simulink model "AbstractFuelControl_M1_FP"  (R2013a)
settings: Solver=ode15s  SolverMode=SingleTasking  StartTime=0  StopTime=simTime  FixedStep=1e-04  RelTol=1e-06  AbsTol=1e-06
values from neighbouring files (symbols this model uses):
  AF_sensor_tol = 1.0    (= 1)    [AbstractFuelControl.m]    (also in AbstractFuelControl_BB.m; AbstractFuelControl_FR.m)
  fault_time = 60    [AbstractFuelControl.m]    (also in AbstractFuelControl_BB.m; AbstractFuelControl_FR.m)
  fuel_inj_tol = 1.0    (= 1)    [AbstractFuelControl.m]    (also in AbstractFuelControl_BB.m; AbstractFuelControl_FR.m)
  MAF_sensor_tol = 1.0    (= 1)    [AbstractFuelControl.m]    (also in AbstractFuelControl_BB.m; AbstractFuelControl_FR.m)
  measureTime = 1    [AbstractFuelControl.m]    (also in AbstractFuelControl_BB.m; AbstractFuelControl_FR.m)
  simTime = 50    [AbstractFuelControl.m]    (also in AbstractFuelControl_BB.m = 15; AbstractFuelControl_FR.m = 12)
  spec_num = 1    [AbstractFuelControl.m]    (also in AbstractFuelControl_BB.m; AbstractFuelControl_FR.m)
(part 1 of 2)
Description:
  | Modeling Engine Timing Using Triggered Subsystems
  | 
  | This example presents a model of a four-cylinder spark ignition engine
  | and demonstrates Simulink(R) capabilities to model an internal combustion
  | engine from the throttle to the crankshaft output. We used well-defined
  | physical principles supplemented, where appropriate, with empirical
  | relationships that describe the systems dynamic behavior without
  | introducing unnecessary complexity.
settings Model: CovMetricSettings=d  ExtModeTrigMode=oneshot  ExtModeArmWhenConnect=off  ExtModeAutoUpdateStatusClock=off  Creator=The MathWorks Inc.  LastModifiedBy=zutshi
settings SolverCC: ConsecutiveZCsStepRelTol=2.8421709430404e-13
settings DataIOCC: ExternalInput=[simTime, en_speed]  InitialState=[]  LimitDataPoints=off  LoadExternalInput=on  SignalLoggingSaveFormat=ModelDataLogs  SaveOutput=off  SignalLogging=off  SaveTime=off  StateSaveName=x  TimeSaveName=t  OutputSaveName=y  SignalLoggingName=sldemo_engine_output
settings OptimizationCC: BlockReduction=off  BooleanDataType=off  ExpressionDepthLimit=2147483647  InitFltsAndDblsToZero=on  OptimizeModelRefInitCode=on  LifeSpan=1  BufferReusableBoundary=off
settings DebuggingCC: SignalInfNanChecking=warning  SaveWithParameterizedLinksMsg=none  SignalResolutionControl=TryResolveAllWithWarning  SolverPrmCheckMsg=none  InheritedTsInSrcMsg=none  MultiTaskDSMMsg=warning  MultiTaskCondExecSysMsg=none  SigSpecEnsureSampleTimeMsg=none  IntegerOverflowMsg=none  ParameterPrecisionLossMsg=none  FcnCallInpInsideContextMsg=UseLocalSettings  UniqueDataStoreMsg=warning  StrictBusMsg=None
settings RTWCC: SystemTargetFile=ert.tlc  TemplateMakefile=ert_default_tmf  Description=Embedded Coder  GenerateReport=on  ProcessScript=ert_make_rtw_hook  IncludeHyperlinkInReport=on  IncludeERTFirstTime=on  GenerateTraceInfo=on  GenerateWebview=on
settings CodeAppCC: IgnoreCustomStorageClasses=off
settings ERTTargetCC: IncludeMdlTerminateFcn=off  MultiInstanceERTCode=on  SupportNonFinite=off  SupportComplex=off  PurelyIntegerCode=on  InlinedParameterPlacement=Hierarchical  ERTCustomFileTemplate=example_file_process.tlc  SuppressUnreachableDefaultCases=on

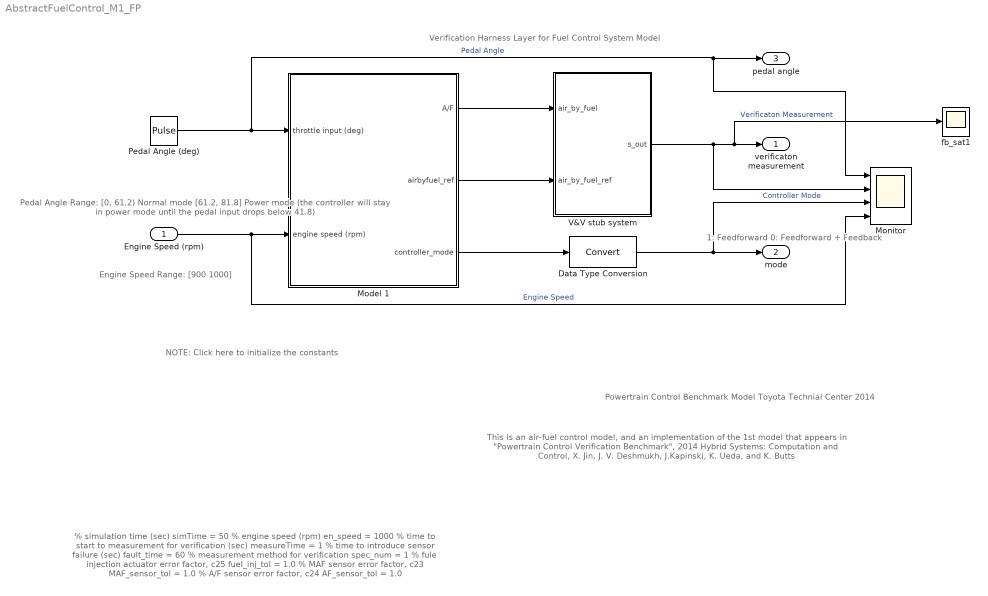
== system AbstractFuelControl_M1_FP ==
  note: 1: Feedforward
      | 0: Feedforward + Feedback
  note: NOTE: Click here to initialize the constants
  note: Pedal Angle Range:
      | [0, 61.2) Normal mode
      | [61.2, 81.8] Power mode (the controller will
      |                    stay in power mode until the pedal
      |                    input drops below 41.8)
  note: This is an air-fuel control model, and an implementation of the 1st model that appears in
      | "Powertrain Control Verification Benchmark", 2014 Hybrid Systems: Computation and Control,
      | X. Jin, J. V. Deshmukh, J.Kapinski, K. Ueda, and K. Butts
  note: % simulation time (sec)
      |     simTime = 50
      | % engine speed (rpm)
      |     en_speed = 1000
      | % time to start to measurement for verification (sec)
      |     measureTime = 1
      | % time to introduce sensor failure (sec)
      |     fault_time = 60
      | % measurement method for verification
      |     spec_num = 1
      | % fule injection actuator error factor, c25
      |     fuel_inj_tol = 1.0
      | % MAF sensor error factor, c23
      |     MAF_sensor_tol = 1.0
      | % A/F sensor error factor, c24
      |     AF_sensor_tol = 1.0
  note: Engine Speed Range:
      | [900 1000]
  note: Powertrain Control Benchmark Model
      | Toyota Technial Center
      | 2014
  note: Verification Harness Layer for Fuel Control System Model
  Engine Speed (rpm) : Inport
  Data Type Conversion : DataTypeConversion
  Model 1 : Subsystem  Priority=1  TreatAsAtomicUnit=on
  "Monitor " : Scope  NumInputPorts=4
      settings: TimeRange=30  YMin=0~-0.15~0~1000  YMax=65~0.175~1~1000
  Pedal Angle (deg) : DiscretePulseGenerator  PulseType=Time based  Amplitude=62  Period=5  PulseWidth=50
  V&V stub system : Subsystem  TreatAsAtomicUnit=on
  fb_sat1 : Scope
      settings: TimeRange=50  YMin=-0.9999  YMax=-0.999899  SaveName=ScopeData26
  verificaton measurement : Outport
  mode : Outport  Port=2
  pedal angle : Outport  Port=3
  wires:
  V&V stub system/1("s_out ") -> "Monitor "/2, fb_sat1/1, verificaton measurement/1  "Verificaton Measurement"
  Model 1/1(A/F) -> V&V stub system/1("air_by_fuel ")
  Engine Speed (rpm)/1 -> "Monitor "/4, Model 1/2(engine speed (rpm))  "Engine Speed"
  Pedal Angle (deg)/1 -> "Monitor "/1, pedal angle/1, Model 1/1(throttle input (deg))  "Pedal Angle"
  Model 1/3(controller_mode) -> Data Type Conversion/1
  Data Type Conversion/1 -> "Monitor "/3, mode/1  "Controller Mode"
  Model 1/2(airbyfuel_ref) -> V&V stub system/2(air_by_fuel_ref)

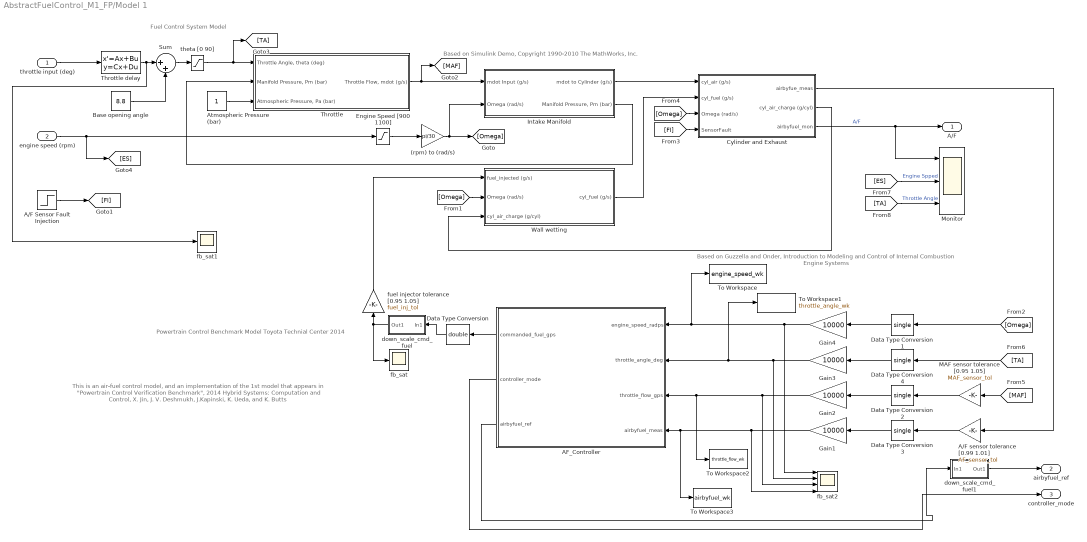
== system AbstractFuelControl_M1_FP/Model 1 ==
  note: Based on Simulink Demo, Copyright 1990-2010 The MathWorks, Inc.
  note: Based on Guzzella and Onder, Introduction to Modeling and Control of Internal Combustion Engine Systems
  note: Fuel Control System Model
  note: This is an air-fuel control model, and an implementation of the 1st model that appears in
      | "Powertrain Control Verification Benchmark", 2014 Hybrid Systems: Computation and Control,
      | X. Jin, J. V. Deshmukh, J.Kapinski, K. Ueda, and K. Butts
  note: Powertrain Control Benchmark Model
      | Toyota Technial Center
      | 2014
  throttle input (deg) : Inport  Description=[0, 81.2]
      settings: AttributesFormatString=%<Description>
  engine speed (rpm) : Inport  Description=[900,1100]  Port=2
      settings: AttributesFormatString=%<Description>
  (rpm) to (rad/s) : Gain  Gain=pi/30
  A/F Sensor Fault Injection : Step  Time=fault_time  SampleTime=0
      settings: AttributesFormatString=1: Failure\n0: Normal
  A/F sensor tolerance [0.99 1.01] : Gain  Gain=AF_sensor_tol
  AF_Controller : Subsystem  TreatAsAtomicUnit=on  SystemSampleTime=0.01
  Atmospheric Pressure (bar) : Constant
  Base opening angle : Constant  Value=8.8
  Cylinder and Exhaust : Subsystem
  Data Type Conversion : DataTypeConversion  OutDataTypeStr=double
  Data Type Conversion{1..4} (4 alike) : DataTypeConversion  OutDataTypeStr=single
  Engine Speed [900 1100] : Saturate  UpperLimit=1100  LowerLimit=900
  Gain1 : Gain  Gain=10000  ParamDataTypeStr=int32  OutDataTypeStr=Inherit: Inherit via back propagation  RndMeth=Simplest  SaturateOnIntegerOverflow=on
      settings: AttributesFormatString=up_scale
  Gain2 : Gain  Gain=10000  ParamDataTypeStr=int32  OutDataTypeStr=int32  RndMeth=Simplest  SaturateOnIntegerOverflow=on
      settings: AttributesFormatString=up_scale
  Gain3 : Gain  Gain=10000  ParamDataTypeStr=int32  OutDataTypeStr=int32  RndMeth=Simplest  SaturateOnIntegerOverflow=on
      settings: AttributesFormatString=up_scale
  Gain4 : Gain  Gain=10000  ParamDataTypeStr=int32  OutDataTypeStr=int32  RndMeth=Simplest  SaturateOnIntegerOverflow=on
      settings: AttributesFormatString=up_scale
  Intake Manifold : Subsystem
  MAF sensor tolerance [0.95 1.05] : Gain  Gain=MAF_sensor_tol
  Monitor : Scope  NumInputPorts=3
      settings: TimeRange=85  YMin=11.75~49.7419~5  YMax=14.75~54.9779~60
  Sum : Sum  Inputs=|++
  Throttle : Subsystem
  Throttle delay : StateSpace  A=-10  C=10  D=0
  To Workspace : ToWorkspace  VariableName=engine_speed_wk  SampleTime=0.01  SaveFormat=Timeseries
  To Workspace1 : ToWorkspace  VariableName=throttle_angle_wk  SampleTime=0.01  SaveFormat=Timeseries
  To Workspace2 : ToWorkspace  VariableName=throttle_flow_wk  SampleTime=0.01  SaveFormat=Timeseries
  To Workspace3 : ToWorkspace  VariableName=airbyfuel_wk  SampleTime=0.01  SaveFormat=Timeseries
  Wall wetting : Subsystem
  down_scale_cmd_fuel : Subsystem
      settings: AttributesFormatString=%<MemberBlocks>
  down_scale_cmd_fuel1 : Subsystem
      settings: AttributesFormatString=%<MemberBlocks>
  fb_sat : Scope
      settings: TimeRange=50  YMin=0.3725  YMax=0.43  SaveName=ScopeData12
  fb_sat1 : Scope
      settings: TimeRange=50  YMin=0.3725  YMax=0.43  SaveName=ScopeData22
  fb_sat2 : Scope  NumInputPorts=4
      settings: TimeRange=0.01302246191310628  YMin=1047196~0~49866.13136574067~0  YMax=1047198~200000~63254.64409722215~200000  SaveName=ScopeData25
  fuel injector tolerance [0.95 1.05] : Gain  Gain=fuel_inj_tol
  theta [0 90] : Saturate  UpperLimit=90  LowerLimit=0
  A/F : Outport
  airbyfuel_ref : Outport  Port=2
  controller_mode : Outport  Port=3
  wires:
  (rpm) to (rad/s)/1 -> [Omega], Intake Manifold/2(Omega (rad/s))
  Data Type Conversion/1 -> down_scale_cmd_fuel/1(In1)
  theta [0 90]/1 -> Throttle/1("Throttle Angle, theta (deg)"), [TA]
  Engine Speed [900 1100]/1 -> (rpm) to (rad/s)/1
  Cylinder and Exhaust/3("airbyfuel_mon ") -> A/F/1, Monitor/1  "A/F"
  Data Type Conversion2/1 -> Gain2/1
  Data Type Conversion3/1 -> Gain1/1
  A/F sensor tolerance [0.99 1.01]/1 -> Data Type Conversion3/1
  [MAF] -> MAF sensor tolerance [0.95 1.05]/1
  Cylinder and Exhaust/1(airbyfue_meas) -> A/F sensor tolerance [0.99 1.01]/1
  Throttle/1("Throttle Flow, mdot (g/s)") -> [MAF], Intake Manifold/1(mdot Input (g/s))
  Intake Manifold/2("Manifold Pressure, Pm (bar)") -> Throttle/2("Manifold Pressure, Pm (bar)")
  Atmospheric Pressure (bar)/1 -> Throttle/3("Atmospheric Pressure, Pa (bar) ")
  Wall wetting/1(cyl_fuel (g/s)) -> Cylinder and Exhaust/2(cyl_fuel (g/s))
  Intake Manifold/1(mdot to Cylinder (g/s)) -> Cylinder and Exhaust/1(cyl_air (g/s))
  [Omega] -> Cylinder and Exhaust/3(Omega (rad/s))
  [Omega] -> Wall wetting/2(Omega (rad/s))
  Cylinder and Exhaust/2(cyl_air_charge (g/cyl)) -> Wall wetting/3(cyl_air_charge (g/cyl))
  [Omega] -> Data Type Conversion1/1
  fuel injector tolerance [0.95 1.05]/1 -> Wall wetting/1(fuel_injected (g/s))
  MAF sensor tolerance [0.95 1.05]/1 -> Data Type Conversion2/1
  Data Type Conversion1/1 -> Gain4/1
  A/F Sensor Fault Injection/1 -> [FI]
  [FI] -> Cylinder and Exhaust/4(SensorFault)
  [TA] -> Data Type Conversion4/1
  Data Type Conversion4/1 -> Gain3/1
  engine speed (rpm)/1 -> [ES], Engine Speed [900 1100]/1
  [TA] -> Monitor/3  "Throttle Angle"
  Base opening angle/1 -> Sum/2
  Sum/1 -> theta [0 90]/1
  AF_Controller/2(controller_mode) -> controller_mode/1
  AF_Controller/3(airbyfuel_ref) -> down_scale_cmd_fuel1/1(In1)
  [ES] -> Monitor/2  "Engine Spped"
  throttle input (deg)/1 -> Throttle delay/1
  Throttle delay/1 -> fb_sat1/1, Sum/1
  AF_Controller/1(commanded_fuel_gps) -> Data Type Conversion/1
  down_scale_cmd_fuel/1(Out1) -> fb_sat/1, fuel injector tolerance [0.95 1.05]/1
  Gain1/1 -> fb_sat2/4, To Workspace3/1, AF_Controller/4(airbyfuel_meas)
  Gain2/1 -> fb_sat2/3, AF_Controller/3(throttle_flow_gps), To Workspace2/1
  Gain3/1 -> fb_sat2/2, To Workspace1/1, AF_Controller/2(throttle_angle_deg)
  Gain4/1 -> To Workspace/1, AF_Controller/1(engine_speed_radps), fb_sat2/1
  down_scale_cmd_fuel1/1(Out1) -> airbyfuel_ref/1

== system AbstractFuelControl_M1_FP/V&V stub system ==
  "air_by_fuel " : Inport  OutDataTypeStr=double
  air_by_fuel_ref : Inport  Port=2
  Calcuate Error : Subsystem  Priority=20  TreatAsAtomicUnit=on
  Constant : Constant  Value=0.5
  Data Type Conversion : DataTypeConversion  OutDataTypeStr=double
  MeasureOn : Step  Time=measureTime  SampleTime=0
  Relational Operator : RelationalOperator  Operator=>  OutDataTypeStr=boolean
  spec_num : Constant  Value=spec_num  OutDataTypeStr=uint8
  "s_out " : Outport
  wires:
  Calcuate Error/1("s_out ") -> "s_out "/1
  MeasureOn/1 -> Relational Operator/1
  Constant/1 -> Relational Operator/2
  Relational Operator/1 -> Calcuate Error/Enable
  spec_num/1 -> Calcuate Error/2(spec_num)
  "air_by_fuel "/1 -> Calcuate Error/1("air_by_fuel ")
  air_by_fuel_ref/1 -> Data Type Conversion/1
  Data Type Conversion/1 -> Calcuate Error/3(air_by_fuel_ref)

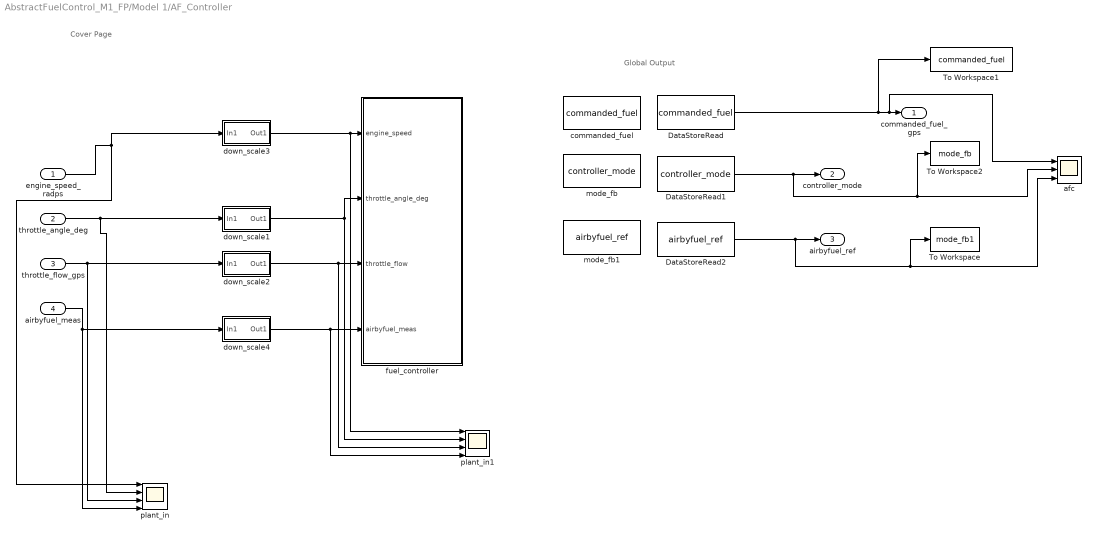
== system AbstractFuelControl_M1_FP/Model 1/AF_Controller ==
  note: Global Output
  note: Cover Page
  engine_speed_radps : Inport
  throttle_angle_deg : Inport  Port=2
  throttle_flow_gps : Inport  Port=3
  airbyfuel_meas : Inport  Port=4
  DataStoreRead : DataStoreRead  Priority=2  DataStoreName=commanded_fuel
  DataStoreRead1 : DataStoreRead  Priority=2  DataStoreName=controller_mode
  DataStoreRead2 : DataStoreRead  Priority=2  DataStoreName=airbyfuel_ref
  To Workspace : ToWorkspace  VariableName=mode_fb1  SampleTime=-1  SaveFormat=Timeseries
  To Workspace1 : ToWorkspace  VariableName=commanded_fuel  SampleTime=-1  SaveFormat=Timeseries
  To Workspace2 : ToWorkspace  VariableName=mode_fb  SampleTime=-1  SaveFormat=Timeseries
  afc : Scope  NumInputPorts=3
      settings: TimeRange=30.1  YMin=16600~-1~147  YMax=16600~1~147  SaveName=ScopeData3
  commanded_fuel : DataStoreMemory  DataStoreName=commanded_fuel  InitialValue=1726
      settings: AttributesFormatString=commanded_fuel
  down_scale1 : Subsystem
      settings: AttributesFormatString=%<MemberBlocks>
  down_scale2 : Subsystem
      settings: AttributesFormatString=%<MemberBlocks>
  down_scale3 : Subsystem
      settings: AttributesFormatString=%<MemberBlocks>
  down_scale4 : Subsystem
      settings: AttributesFormatString=%<MemberBlocks>
  fuel_controller : Subsystem  Priority=1  TreatAsAtomicUnit=on
      settings: AttributesFormatString=Priority = %<Priority>
  mode_fb : DataStoreMemory  DataStoreName=controller_mode  InitialValue=1  OutDataTypeStr=boolean
      settings: AttributesFormatString=controller_mode
  mode_fb1 : DataStoreMemory  DataStoreName=airbyfuel_ref  InitialValue=147  OutDataTypeStr=single
  plant_in : Scope  NumInputPorts=4
      settings: TimeRange=30.1  YMin=99.484~8~5~-5  YMax=109.956~19~8.25~5  SaveName=ScopeData10
  plant_in1 : Scope  NumInputPorts=4
      settings: TimeRange=30.1  YMin=98.8~8~4.75~-5  YMax=109.2~18~5.25~5  SaveName=ScopeData11
  commanded_fuel_gps : Outport
  controller_mode : Outport  Port=2
  airbyfuel_ref : Outport  Port=3
  wires:
  DataStoreRead2/1 -> To Workspace/1, afc/3, airbyfuel_ref/1
  DataStoreRead1/1 -> To Workspace2/1, afc/2, controller_mode/1
  airbyfuel_meas/1 -> down_scale4/1(In1), plant_in/4
  throttle_flow_gps/1 -> down_scale2/1(In1), plant_in/3
  throttle_angle_deg/1 -> down_scale1/1(In1), plant_in/2
  engine_speed_radps/1 -> down_scale3/1(In1), plant_in/1
  DataStoreRead/1 -> To Workspace1/1, afc/1, commanded_fuel_gps/1
  down_scale2/1(Out1) -> plant_in1/3, fuel_controller/3(throttle_flow)
  down_scale1/1(Out1) -> fuel_controller/2(throttle_angle_deg), plant_in1/2
  down_scale3/1(Out1) -> plant_in1/1, fuel_controller/1(engine_speed)
  down_scale4/1(Out1) -> plant_in1/4, fuel_controller/4(airbyfuel_meas)

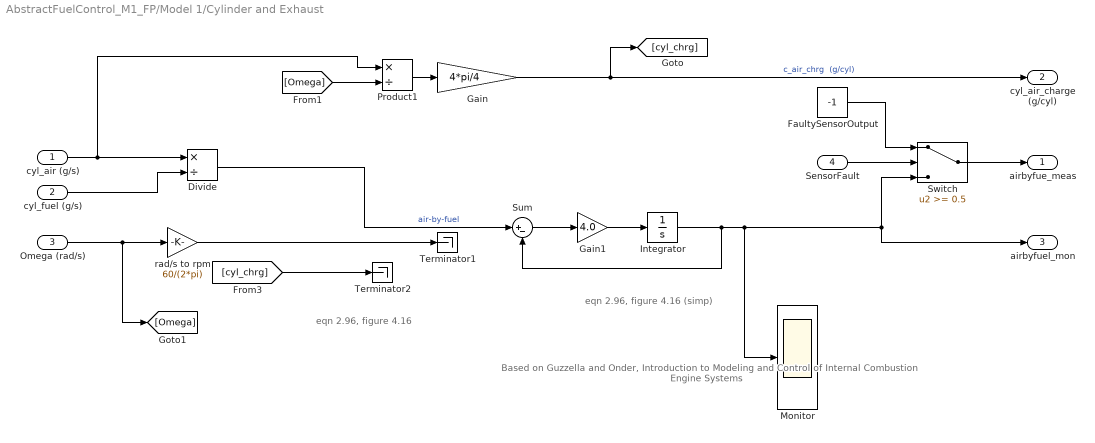
== system AbstractFuelControl_M1_FP/Model 1/Cylinder and Exhaust ==
  note: Based on Guzzella and Onder, Introduction to Modeling and Control of Internal Combustion Engine Systems
  note: eqn 2.96, figure 4.16
  note: eqn 2.96, figure 4.16 (simp)
  cyl_air (g/s) : Inport
  cyl_fuel (g/s) : Inport  Port=2
  Omega (rad/s) : Inport  Port=3
  SensorFault : Inport  Port=4
  Divide : Product  Inputs=*/
  FaultySensorOutput : Constant  Value=-1
  Gain : Gain  Gain=4*pi/4
  Gain1 : Gain  Gain=4.0
  Integrator : Integrator  ContinuousStateAttributes='cyl_ex'
  Monitor : Scope
      settings: TimeRange=85  YMin=11.75  YMax=14.75  SaveName=ScopeData21
  Product1 : Product  Inputs=*/  RndMeth=Zero
  Sum : Sum  Inputs=|+-
  Switch : Switch  Threshold=0.5
  Terminator1 : Terminator
  Terminator2 : Terminator
  rad/s to rpm : Gain  Gain=60/(2*pi)
  airbyfue_meas : Outport
  cyl_air_charge (g/cyl) : Outport  Port=2
  "airbyfuel_mon " : Outport  Port=3
  wires:
  cyl_air (g/s)/1 -> Divide/1, Product1/1
  [Omega] -> Product1/2
  Product1/1 -> Gain/1
  Gain/1 -> [cyl_chrg], cyl_air_charge (g/cyl)/1  "c_air_chrg  (g/cyl)"
  cyl_fuel (g/s)/1 -> Divide/2
  Omega (rad/s)/1 -> [Omega], rad/s to rpm/1
  Switch/1 -> airbyfue_meas/1
  FaultySensorOutput/1 -> Switch/1
  SensorFault/1 -> Switch/2
  Integrator/1 -> Monitor/1, "airbyfuel_mon "/1, Switch/3, Sum/2
  Divide/1 -> Sum/1  "air-by-fuel"
  rad/s to rpm/1 -> Terminator1/1
  [cyl_chrg] -> Terminator2/1
  Gain1/1 -> Integrator/1
  Sum/1 -> Gain1/1

== system AbstractFuelControl_M1_FP/Model 1/Intake Manifold ==
  note: Intake Manifold Vacuum
  note: Based on Simulink Demo, Copyright 1990-2010 The MathWorks, Inc.
  mdot Input (g/s) : Inport
  Omega (rad/s) : Inport  Port=2
  Gain2 : Gain  Gain=0.9  ParamDataTypeStr=single  OutDataTypeStr=Inherit: Inherit via back propagation  RndMeth=Simplest  SaturateOnIntegerOverflow=on
      settings: AttributesFormatString=pumping tolerance [0.9 1.1]
  Mux : Mux  Inputs=2
  Pumping : Fcn  Expr=-0.366 + 0.08979*u[1]*u[2] - 0.0337*u[2]*u[1]*u[1] + 0.0001*u[1]*u[2]*u[2]
  RT/Vm : Gain  Gain=0.41328  SaturateOnIntegerOverflow=on  OutDataTypeStr=Inherit: Same as input  ParamDataTypeStr=Inherit: Same as input
  Sum : Sum  Inputs=|+-  SaturateOnIntegerOverflow=on  InputSameDT=on  OutDataTypeStr=Inherit: Same as first input
  fb_sat1 : Scope
      settings: TimeRange=50  YMin=0.3725  YMax=0.43  SaveName=ScopeData23
  p0 = 0.543 (bar) : Integrator  InitialCondition=0.982  ContinuousStateAttributes='intake_manifold'
  mdot to Cylinder (g/s) : Outport  InitialOutput=0
  "Manifold Pressure, Pm (bar)" : Outport  Port=2  InitialOutput=0
  wires:
  mdot Input (g/s)/1 -> Sum/1
  RT/Vm/1 -> p0 = 0.543 (bar)/1
  Omega (rad/s)/1 -> Mux/2
  Mux/1 -> Pumping/1
  p0 = 0.543 (bar)/1 -> fb_sat1/1, Mux/1, "Manifold Pressure, Pm (bar)"/1
  Sum/1 -> RT/Vm/1
  Pumping/1 -> Gain2/1
  Gain2/1 -> Sum/2, mdot to Cylinder (g/s)/1

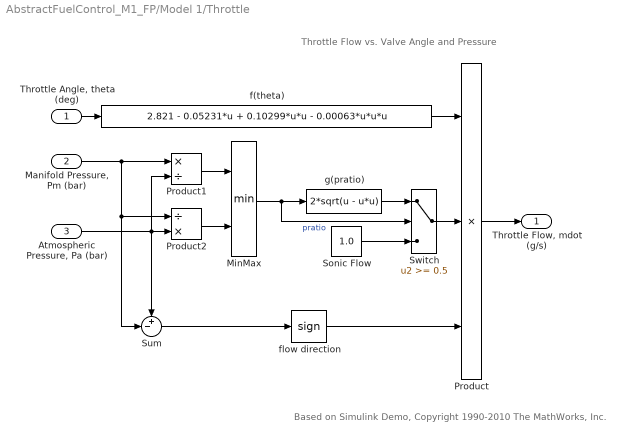
== system AbstractFuelControl_M1_FP/Model 1/Throttle ==
  note: Throttle Flow vs. Valve Angle and Pressure
  note: Based on Simulink Demo, Copyright 1990-2010 The MathWorks, Inc.
  "Throttle Angle, theta (deg)" : Inport
  "Manifold Pressure, Pm (bar)" : Inport  Port=2
  "Atmospheric Pressure, Pa (bar) " : Inport  Port=3
  MinMax : MinMax  Inputs=2  SaturateOnIntegerOverflow=on  InputSameDT=on
  Product : Product  Inputs=3  SaturateOnIntegerOverflow=on  RndMeth=Zero  InputSameDT=on  OutDataTypeStr=Inherit: Same as first input
  Product1 : Product  Inputs=*/  SaturateOnIntegerOverflow=on  RndMeth=Zero  InputSameDT=on  OutDataTypeStr=Inherit: Same as first input
  Product2 : Product  Inputs=/*  SaturateOnIntegerOverflow=on  RndMeth=Zero  InputSameDT=on  OutDataTypeStr=Inherit: Same as first input
  "Sonic Flow " : Constant  Value=1.0
  Sum : Sum  Inputs=+-|  SaturateOnIntegerOverflow=on  InputSameDT=on  OutDataTypeStr=Inherit: Same as first input
  Switch : Switch  Threshold=0.5  SaturateOnIntegerOverflow=on  InputSameDT=on
  f(theta) : Fcn  Expr=2.821 - 0.05231*u + 0.10299*u*u - 0.00063*u*u*u
  flow direction : Signum
  g(pratio) : Fcn  Expr=2*sqrt(u - u*u)
  "Throttle Flow, mdot (g/s)" : Outport  InitialOutput=0
  wires:
  "Manifold Pressure, Pm (bar)"/1 -> Sum/2, Product2/1, Product1/1
  Product2/1 -> MinMax/2
  Product1/1 -> MinMax/1
  "Atmospheric Pressure, Pa (bar) "/1 -> Sum/1, Product2/2, Product1/2
  g(pratio)/1 -> Switch/1
  "Sonic Flow "/1 -> Switch/3
  Switch/1 -> Product/2
  flow direction/1 -> Product/3
  Sum/1 -> flow direction/1
  MinMax/1 -> g(pratio)/1, Switch/2  "pratio"
  "Throttle Angle, theta (deg)"/1 -> f(theta)/1
  Product/1 -> "Throttle Flow, mdot (g/s)"/1
  f(theta)/1 -> Product/1

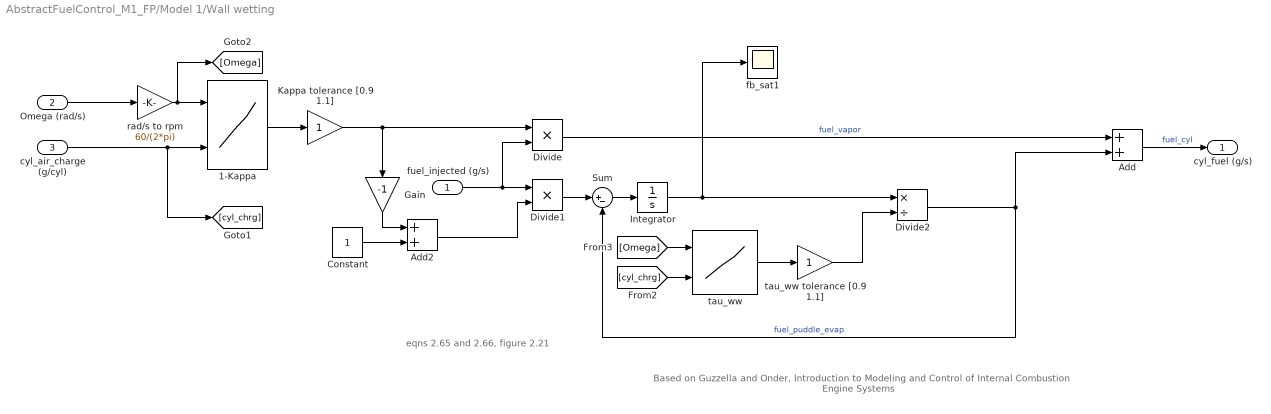
== system AbstractFuelControl_M1_FP/Model 1/Wall wetting ==
  note: Based on Guzzella and Onder, Introduction to Modeling and Control of Internal Combustion Engine Systems
  note: eqns 2.65 and 2.66, figure 2.21
  fuel_injected (g/s) : Inport
  Omega (rad/s) : Inport  Port=2
  cyl_air_charge (g/cyl) : Inport  Port=3
  1-Kappa : Lookup_n-D  BreakpointsForDimension1=[1000,1500,2000,2500,3000]  BreakpointsForDimension2=[.1,.2,.3,.4]  Table=reshape([0.8,.7,.7,.8,.9,.7,.66,.65,.73,.85,.66,.66,.63,.66,.8,.6,.6,.6,.6,.7],5,4)  UseLastTableValue=on  RndMeth=Simplest  InputSameDT=on
  Add : Sum
  Add2 : Sum
  Constant : Constant
  Divide : Product  Inputs=**
  Divide1 : Product  Inputs=**
  Divide2 : Product  Inputs=*/
  Gain : Gain  Gain=-1
  Integrator : Integrator  InitialCondition=0.0112  ContinuousStateAttributes='wall_wetting'
  Kappa tolerance [0.9 1.1] : Gain
  Sum : Sum  Inputs=|+-
  fb_sat1 : Scope
      settings: TimeRange=50  YMin=0.3725  YMax=0.43  SaveName=ScopeData24
  rad/s to rpm : Gain  Gain=60/(2*pi)
  tau_ww : Lookup_n-D  BreakpointsForDimension1=[1000,1500,2000,2500,3000]  BreakpointsForDimension2=[0.1,0.2,0.3,0.4]  Table=reshape([.4,.3,.35,.3,.2,.22,.22,.4,.35,.5,.20,.22,.5,.4,.35,.35,.3,.45,.5,.4],5,4)  UseLastTableValue=on  RndMeth=Simplest  InputSameDT=on
  tau_ww tolerance [0.9 1.1] : Gain
  cyl_fuel (g/s) : Outport
  wires:
  1-Kappa/1 -> Kappa tolerance [0.9 1.1]/1
  fuel_injected (g/s)/1 -> Divide/2, Divide1/1
  Divide/1 -> Add/1  "fuel_vapor"
  Add/1 -> cyl_fuel (g/s)/1  "fuel_cyl"
  Integrator/1 -> fb_sat1/1, Divide2/1
  Divide1/1 -> Sum/1
  Sum/1 -> Integrator/1
  Divide2/1 -> Add/2, Sum/2  "fuel_puddle_evap"
  Add2/1 -> Divide1/2
  cyl_air_charge (g/cyl)/1 -> 1-Kappa/2, [cyl_chrg]
  [cyl_chrg] -> tau_ww/2
  tau_ww/1 -> tau_ww tolerance [0.9 1.1]/1
  Gain/1 -> Add2/1
  Constant/1 -> Add2/2
  rad/s to rpm/1 -> [Omega], 1-Kappa/1
  Omega (rad/s)/1 -> rad/s to rpm/1
  Kappa tolerance [0.9 1.1]/1 -> Divide/1, Gain/1
  tau_ww tolerance [0.9 1.1]/1 -> Divide2/2
  [Omega] -> tau_ww/1

== system AbstractFuelControl_M1_FP/Model 1/down_scale_cmd_fuel ==
  In1 : Inport
  Constant8 : Constant  Value=10000  OutDataTypeStr=single  SampleTime=-1
      settings: AttributesFormatString=Value = %<Value>
  Divide2 : Product  Inputs=*/  OutDataTypeStr=Inherit: Inherit via back propagation
  Out1 : Outport
  wires:
  Constant8/1 -> Divide2/2
  Divide2/1 -> Out1/1
  In1/1 -> Divide2/1

== system AbstractFuelControl_M1_FP/Model 1/down_scale_cmd_fuel1 ==
  In1 : Inport
  Constant8 : Constant  Value=10  OutDataTypeStr=single  SampleTime=-1
      settings: AttributesFormatString=Value = %<Value>
  Divide2 : Product  Inputs=*/  OutDataTypeStr=Inherit: Inherit via back propagation
  Out1 : Outport
  wires:
  Constant8/1 -> Divide2/2
  Divide2/1 -> Out1/1
  In1/1 -> Divide2/1

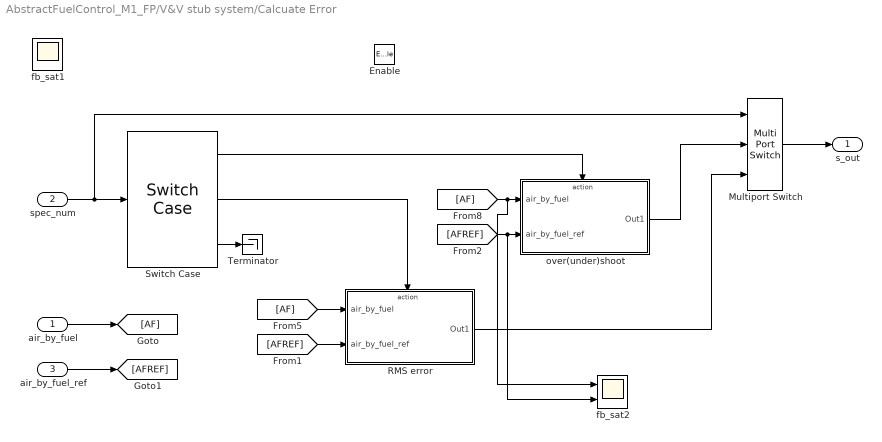
== system AbstractFuelControl_M1_FP/V&V stub system/Calcuate Error ==
  "air_by_fuel " : Inport
  spec_num : Inport  Port=2  OutDataTypeStr=uint8
  air_by_fuel_ref : Inport  Port=3
  Enable : EnablePort
  Multiport Switch : MultiPortSwitch  Inputs=2
  RMS error : Subsystem  TreatAsAtomicUnit=on
  Switch Case : SwitchCase  CaseConditions={1,2}
  Terminator : Terminator
  fb_sat1 : Scope
      settings: TimeRange=50  YMin=-0.9999  YMax=-0.999899  SaveName=ScopeData27
  fb_sat2 : Scope  NumInputPorts=2
      settings: TimeRange=50  YMin=14.425~147000  YMax=14.925~147000  SaveName=ScopeData28
  over(under)shoot : Subsystem  TreatAsAtomicUnit=on
  "s_out " : Outport
  wires:
  "air_by_fuel "/1 -> [AF]
  spec_num/1 -> Multiport Switch/1, Switch Case/1
  Switch Case/1 -> over(under)shoot/Action
  [AF] -> fb_sat2/1, over(under)shoot/1("air_by_fuel ")
  Switch Case/2 -> RMS error/Action
  [AF] -> RMS error/1("air_by_fuel ")
  Multiport Switch/1 -> "s_out "/1
  over(under)shoot/1(Out1) -> Multiport Switch/2
  RMS error/1(Out1) -> Multiport Switch/3
  Switch Case/3 -> Terminator/1
  air_by_fuel_ref/1 -> [AFREF]
  [AFREF] -> RMS error/2(air_by_fuel_ref)
  [AFREF] -> fb_sat2/2, over(under)shoot/2(air_by_fuel_ref)

== system AbstractFuelControl_M1_FP/Model 1/AF_Controller/down_scale1 ==
  In1 : Inport
  Constant8 : Constant  Value=1000  OutDataTypeStr=single  SampleTime=-1
      settings: AttributesFormatString=Value = %<Value>
  Divide2 : Product  Inputs=*/  OutDataTypeStr=Inherit: Inherit via back propagation
  Out1 : Outport
  wires:
  Constant8/1 -> Divide2/2
  Divide2/1 -> Out1/1
  In1/1 -> Divide2/1

== system AbstractFuelControl_M1_FP/Model 1/AF_Controller/down_scale2 ==
  In1 : Inport
  Constant8 : Constant  Value=1000  OutDataTypeStr=single  SampleTime=-1
      settings: AttributesFormatString=Value = %<Value>
  Divide2 : Product  Inputs=*/  OutDataTypeStr=Inherit: Inherit via back propagation
  Out1 : Outport
  wires:
  Constant8/1 -> Divide2/2
  Divide2/1 -> Out1/1
  In1/1 -> Divide2/1

== system AbstractFuelControl_M1_FP/Model 1/AF_Controller/down_scale3 ==
  In1 : Inport
  Constant8 : Constant  Value=1000  OutDataTypeStr=single  SampleTime=-1
      settings: AttributesFormatString=Value = %<Value>
  Divide2 : Product  Inputs=*/  OutDataTypeStr=Inherit: Inherit via back propagation
  Out1 : Outport
  wires:
  Constant8/1 -> Divide2/2
  Divide2/1 -> Out1/1
  In1/1 -> Divide2/1

== system AbstractFuelControl_M1_FP/Model 1/AF_Controller/down_scale4 ==
  In1 : Inport
  Constant8 : Constant  Value=1000  OutDataTypeStr=single  SampleTime=-1
      settings: AttributesFormatString=Value = %<Value>
  Divide2 : Product  Inputs=*/  OutDataTypeStr=Inherit: Inherit via back propagation
  Out1 : Outport
  wires:
  Constant8/1 -> Divide2/2
  Divide2/1 -> Out1/1
  In1/1 -> Divide2/1

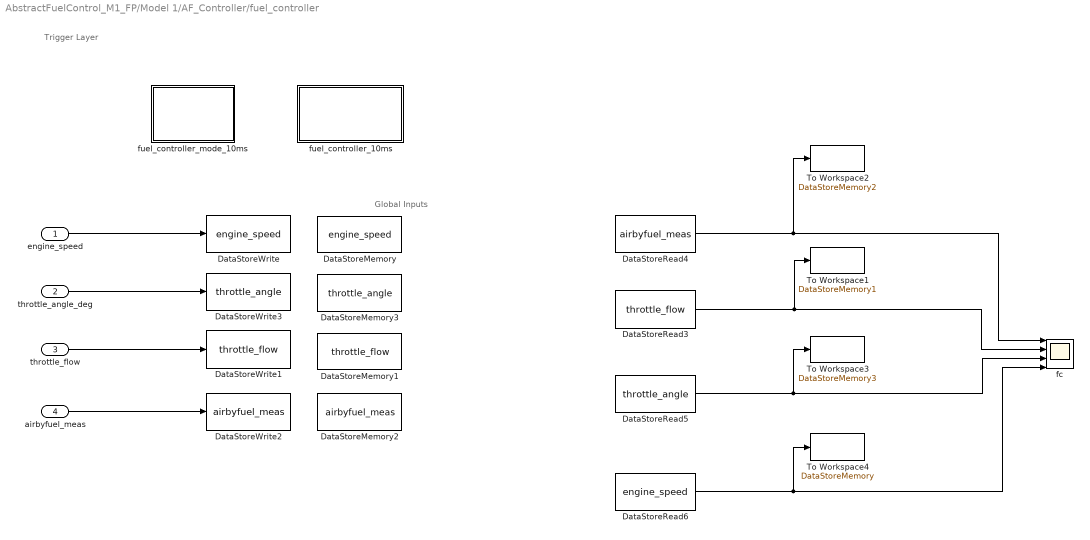
== system AbstractFuelControl_M1_FP/Model 1/AF_Controller/fuel_controller ==
  note: Global Inputs
  note: Trigger Layer
  engine_speed : Inport
  throttle_angle_deg : Inport  Port=2
  throttle_flow : Inport  Port=3
  airbyfuel_meas : Inport  Port=4
  DataStoreMemory : DataStoreMemory  DataStoreName=engine_speed  OutDataTypeStr=single
      settings: AttributesFormatString=engine speed
  DataStoreMemory1 : DataStoreMemory  DataStoreName=throttle_flow  OutDataTypeStr=single
      settings: AttributesFormatString=throttle flow
  DataStoreMemory2 : DataStoreMemory  DataStoreName=airbyfuel_meas  OutDataTypeStr=single
      settings: AttributesFormatString=lambda_meas
  DataStoreMemory3 : DataStoreMemory  DataStoreName=throttle_angle  OutDataTypeStr=single
      settings: AttributesFormatString=throttle flow
  DataStoreRead3 : DataStoreRead  DataStoreName=throttle_flow
  DataStoreRead4 : DataStoreRead  DataStoreName=airbyfuel_meas
  DataStoreRead5 : DataStoreRead  DataStoreName=throttle_angle
  DataStoreRead6 : DataStoreRead  DataStoreName=engine_speed
  DataStoreWrite : DataStoreWrite  Priority=1  DataStoreName=engine_speed
  DataStoreWrite1 : DataStoreWrite  Priority=1  DataStoreName=throttle_flow
  DataStoreWrite2 : DataStoreWrite  Priority=1  DataStoreName=airbyfuel_meas
  DataStoreWrite3 : DataStoreWrite  Priority=1  DataStoreName=throttle_angle
  To Workspace1 : ToWorkspace  VariableName=DataStoreMemory1  SampleTime=-1  SaveFormat=Timeseries
      settings: MaxDataPoints=1
  To Workspace2 : ToWorkspace  VariableName=DataStoreMemory2  SampleTime=-1  SaveFormat=Timeseries
      settings: MaxDataPoints=1
  To Workspace3 : ToWorkspace  VariableName=DataStoreMemory3  SampleTime=-1  SaveFormat=Timeseries
      settings: MaxDataPoints=1
  To Workspace4 : ToWorkspace  VariableName=DataStoreMemory  SampleTime=-1  SaveFormat=Timeseries
      settings: MaxDataPoints=1
  fc : Scope  NumInputPorts=4
      settings: TimeRange=30.1  YMin=14.5~5.5~8~99.484  YMax=15.1~8.5~19~109.956
  fuel_controller_10ms : Subsystem  Priority=30  TreatAsAtomicUnit=on
      settings: AttributesFormatString=Priority = %<Priority>
  fuel_controller_mode_10ms : Subsystem  Priority=20  TreatAsAtomicUnit=on
      settings: AttributesFormatString=Priority = %<Priority>
  wires:
  DataStoreRead4/1 -> To Workspace2/1, fc/1
  DataStoreRead3/1 -> To Workspace1/1, fc/2
  DataStoreRead5/1 -> To Workspace3/1, fc/3
  DataStoreRead6/1 -> To Workspace4/1, fc/4
  engine_speed/1 -> DataStoreWrite/1
  throttle_angle_deg/1 -> DataStoreWrite3/1
  throttle_flow/1 -> DataStoreWrite1/1
  airbyfuel_meas/1 -> DataStoreWrite2/1

== system AbstractFuelControl_M1_FP/V&V stub system/Calcuate Error/RMS error ==
  "air_by_fuel " : Inport
  air_by_fuel_ref : Inport  Port=2
  Action Port : ActionPort  ActionType=case
  Constant : Constant  Value=simTime-10
  Divide : Product  Inputs=*/
  Integrator : Integrator  ContinuousStateAttributes='vnv'
  Math Function : Math  Operator=square  SaturateOnIntegerOverflow=on
  MeasureOn : Step  Time=10  SampleTime=0
  Product : Product
  Sqrt : Sqrt  SaturateOnIntegerOverflow=on
  Sum1 : Sum  Inputs=+-  OutDataTypeStr=Inherit: Inherit via back propagation  RndMeth=Simplest  InputSameDT=on
  Out1 : Outport
  wires:
  Sum1/1 -> Math Function/1
  Math Function/1 -> Product/1
  "air_by_fuel "/1 -> Sum1/1
  Divide/1 -> Sqrt/1
  Constant/1 -> Divide/2
  air_by_fuel_ref/1 -> Sum1/2
  MeasureOn/1 -> Product/2
  Product/1 -> Integrator/1
  Integrator/1 -> Divide/1
  Sqrt/1 -> Out1/1

== system AbstractFuelControl_M1_FP/V&V stub system/Calcuate Error/over(under)shoot ==
  "air_by_fuel " : Inport
  air_by_fuel_ref : Inport  Port=2
  Action Port : ActionPort  ActionType=case
  Constant : Constant
  Divide : Product  Inputs=*/
  Sum1 : Sum  Inputs=+-  OutDataTypeStr=Inherit: Inherit via back propagation  RndMeth=Simplest  InputSameDT=on
  Out1 : Outport
  wires:
  "air_by_fuel "/1 -> Divide/1
  Divide/1 -> Sum1/1
  Constant/1 -> Sum1/2
  Sum1/1 -> Out1/1
  air_by_fuel_ref/1 -> Divide/2

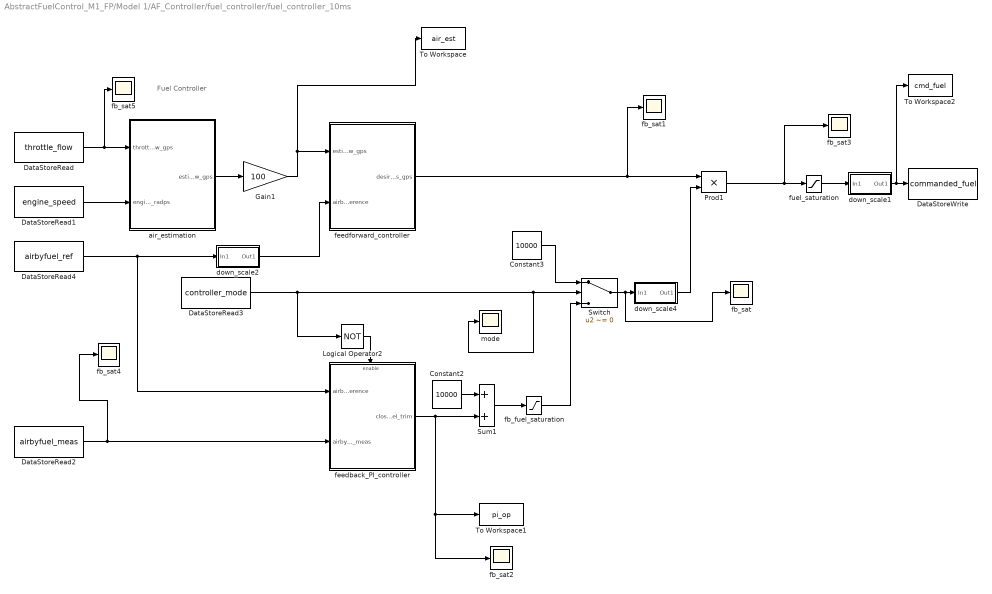
== system AbstractFuelControl_M1_FP/Model 1/AF_Controller/fuel_controller/fuel_controller_10ms ==
  note: Fuel Controller
  Constant2 : Constant  Value=10000  OutDataTypeStr=Inherit: Inherit via back propagation
  Constant3 : Constant  Value=10000  OutDataTypeStr=Inherit: Inherit via back propagation
  DataStoreRead : DataStoreRead  DataStoreName=throttle_flow
  DataStoreRead1 : DataStoreRead  DataStoreName=engine_speed
  DataStoreRead2 : DataStoreRead  DataStoreName=airbyfuel_meas
  DataStoreRead3 : DataStoreRead  DataStoreName=controller_mode
      settings: AttributesFormatString=1: Feedforward\n0: Feedforward + Feedback
  DataStoreRead4 : DataStoreRead  DataStoreName=airbyfuel_ref
  DataStoreWrite : DataStoreWrite  DataStoreName=commanded_fuel
  Gain1 : Gain  Gain=100  OutDataTypeStr=Inherit: Inherit via back propagation  ParamDataTypeStr=Inherit: Same as input
      settings: AttributesFormatString=up_scale
  Logical Operator2 : Logic  Operator=NOT  AllPortsSameDT=off  OutDataTypeStr=boolean
  Prod1 : Product  OutDataTypeStr=single
  Sum1 : Sum  AccumDataTypeStr=single  OutDataTypeStr=single  InputSameDT=on
  Switch : Switch  Criteria=u2 ~= 0  Threshold=0.5  OutDataTypeStr=single  ZeroCross=off
  To Workspace : ToWorkspace  VariableName=air_est  SampleTime=-1  SaveFormat=Timeseries
  To Workspace1 : ToWorkspace  VariableName=pi_op  SampleTime=-1  SaveFormat=Timeseries
  To Workspace2 : ToWorkspace  VariableName=cmd_fuel  SampleTime=-1  SaveFormat=Timeseries
  air_estimation : Subsystem  TreatAsAtomicUnit=on
  down_scale1 : Subsystem
      settings: AttributesFormatString=%<MemberBlocks>
  down_scale2 : Subsystem
      settings: AttributesFormatString=%<MemberBlocks>
  down_scale4 : Subsystem
      settings: AttributesFormatString=%<MemberBlocks>
  fb_fuel_saturation : Saturate  UpperLimit=2147483647  LowerLimit=0  LinearizeAsGain=off  ZeroCross=off  OutDataTypeStr=single  RndMeth=Round
      settings: AttributesFormatString=y >= 0
  fb_sat{,1..5} (6 alike) : Scope
      fb_sat settings: TimeRange=50  YMin=0  YMax=2000000  SaveName=ScopeData4
      fb_sat1 settings: TimeRange=30.1  YMin=2.85  YMax=3.15  SaveName=ScopeData5
      fb_sat2 settings: TimeRange=30.1  YMin=-4.5  YMax=3.5  SaveName=ScopeData7
      fb_sat3 settings: TimeRange=30.1  YMin=3800  YMax=4450  SaveName=ScopeData8
      fb_sat4 settings: TimeRange=30.1  YMin=5.575  YMax=6  SaveName=ScopeData9
      fb_sat5 settings: TimeRange=30.1  YMin=25  YMax=82.5  SaveName=ScopeData17
  feedback_PI_controller : Subsystem  TreatAsAtomicUnit=on
  feedforward_controller : Subsystem  TreatAsAtomicUnit=on
  fuel_saturation : Saturate  UpperLimit=1660000  LowerLimit=130000  LinearizeAsGain=off  ZeroCross=off  OutDataTypeStr=single
      settings: AttributesFormatString=0.13 <=\ncommanded_fuel\n<= 1.66
  mode : Scope
      settings: TimeRange=30.1  YMin=0.994  YMax=1.006  SaveName=ScopeData6
  wires:
  DataStoreRead4/1 -> feedback_PI_controller/1(airbyfuel_reference), down_scale2/1(In1)
  feedback_PI_controller/1(closed_loop_fuel_trim) -> fb_sat2/1, To Workspace1/1, Sum1/2
  Constant2/1 -> Sum1/1
  air_estimation/1(estimated_cyl_air_flow_gps) -> Gain1/1
  DataStoreRead1/1 -> air_estimation/2(engine_speed_radps)
  DataStoreRead/1 -> fb_sat5/1, air_estimation/1(throttle_flow_gps)
  Sum1/1 -> fb_fuel_saturation/1
  DataStoreRead3/1 -> Logical Operator2/1, mode/1, Switch/2
  Constant3/1 -> Switch/1
  fb_fuel_saturation/1 -> Switch/3
  Logical Operator2/1 -> feedback_PI_controller/Enable
  DataStoreRead2/1 -> fb_sat4/1, feedback_PI_controller/2(airbyfuel_meas)
  Gain1/1 -> To Workspace/1, feedforward_controller/1(estimated_cyl_air_flow_gps)
  Switch/1 -> fb_sat/1, down_scale4/1(In1)
  fuel_saturation/1 -> down_scale1/1(In1)
  feedforward_controller/1(desired_fuel_mass_gps) -> Prod1/1, fb_sat1/1
  down_scale4/1(Out1) -> Prod1/2
  down_scale1/1(Out1) -> DataStoreWrite/1, To Workspace2/1
  down_scale2/1(Out1) -> feedforward_controller/2(airbyfuel_reference)
  Prod1/1 -> fb_sat3/1, fuel_saturation/1

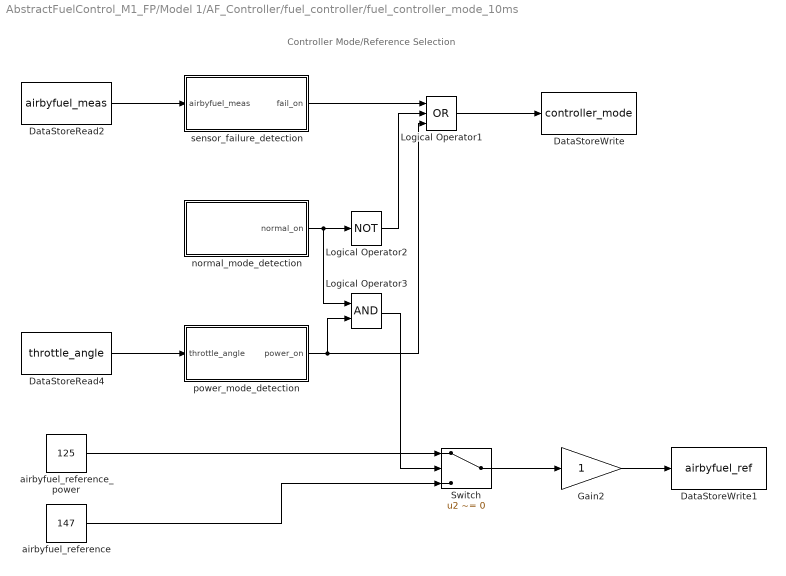
== system AbstractFuelControl_M1_FP/Model 1/AF_Controller/fuel_controller/fuel_controller_mode_10ms ==
  note: Controller Mode/Reference Selection
  DataStoreRead2 : DataStoreRead  DataStoreName=airbyfuel_meas
  DataStoreRead4 : DataStoreRead  DataStoreName=throttle_angle
  DataStoreWrite : DataStoreWrite  DataStoreName=controller_mode
      settings: AttributesFormatString=1: Feedforward\n0: Feedforward + Feedback
  DataStoreWrite1 : DataStoreWrite  DataStoreName=airbyfuel_ref
  Gain2 : Gain  ParamDataTypeStr=fixdt(1,32,30)  OutDataTypeStr=Inherit: Inherit via back propagation  RndMeth=Simplest  SaturateOnIntegerOverflow=on
      settings: AttributesFormatString=up_scale
  Logical Operator1 : Logic  Operator=OR  Inputs=3  AllPortsSameDT=off  OutDataTypeStr=boolean
  Logical Operator2 : Logic  Operator=NOT  AllPortsSameDT=off  OutDataTypeStr=boolean
  Logical Operator3 : Logic  AllPortsSameDT=off  OutDataTypeStr=boolean
  Switch : Switch  Criteria=u2 ~= 0  OutDataTypeStr=Inherit: Inherit via back propagation
  airbyfuel_reference : Constant  Value=147  OutDataTypeStr=Inherit: Inherit via back propagation  SampleTime=-1
  airbyfuel_reference_power : Constant  Value=125  OutDataTypeStr=Inherit: Inherit via back propagation  SampleTime=-1
  normal_mode_detection : Subsystem  TreatAsAtomicUnit=on
      settings: AttributesFormatString=0: Feedforward\n1: Feedforward + Feedback
  power_mode_detection : Subsystem  TreatAsAtomicUnit=on
      settings: AttributesFormatString=1: Feedforward\n0: Feedforward + Feedback
  sensor_failure_detection : Subsystem  TreatAsAtomicUnit=on
      settings: AttributesFormatString=1: Feedforward\n0: Feedforward + Feedback
  wires:
  sensor_failure_detection/1(fail_on) -> Logical Operator1/1
  DataStoreRead4/1 -> power_mode_detection/1(throttle_angle)
  DataStoreRead2/1 -> sensor_failure_detection/1(airbyfuel_meas)
  Logical Operator1/1 -> DataStoreWrite/1
  normal_mode_detection/1(normal_on) -> Logical Operator3/1, Logical Operator2/1
  Switch/1 -> Gain2/1
  power_mode_detection/1(power_on) -> Logical Operator3/2, Logical Operator1/3
  Logical Operator2/1 -> Logical Operator1/2
  airbyfuel_reference_power/1 -> Switch/1
  airbyfuel_reference/1 -> Switch/3
  Logical Operator3/1 -> Switch/2
  Gain2/1 -> DataStoreWrite1/1

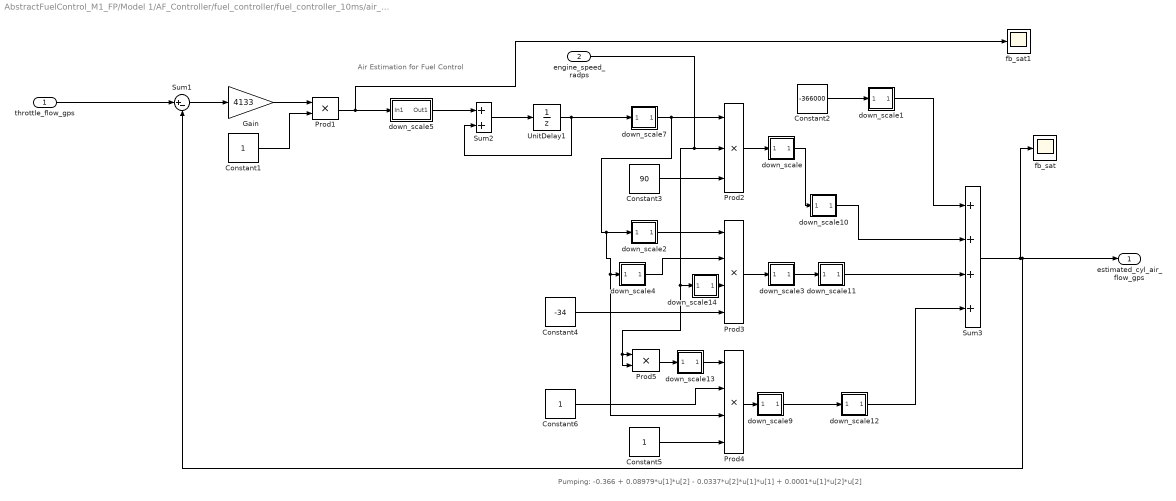
== system AbstractFuelControl_M1_FP/Model 1/AF_Controller/fuel_controller/fuel_controller_10ms/air_estimation ==
  note: Air Estimation for Fuel Control
  note: Pumping: -0.366 + 0.08979*u[1]*u[2] - 0.0337*u[2]*u[1]*u[1] + 0.0001*u[1]*u[2]*u[2]
  throttle_flow_gps : Inport
  engine_speed_radps : Inport  Port=2
  Constant1 : Constant  OutDataTypeStr=Inherit: Inherit via back propagation  SampleTime=-1
      settings: AttributesFormatString=Sample Time (s)
  Constant2 : Constant  Value=-366000  OutDataTypeStr=Inherit: Inherit via back propagation  SampleTime=-1
  Constant3 : Constant  Value=90  OutDataTypeStr=Inherit: Inherit via back propagation  SampleTime=-1
  Constant4 : Constant  Value=-34  OutDataTypeStr=single  SampleTime=-1
  Constant5 : Constant  OutDataTypeStr=Inherit: Inherit via back propagation  SampleTime=-1
  Constant6 : Constant  OutDataTypeStr=Inherit: Inherit via back propagation  SampleTime=-1
  Gain : Gain  Gain=4133  OutDataTypeStr=Inherit: Inherit via back propagation  RndMeth=Simplest  SaturateOnIntegerOverflow=on  ParamDataTypeStr=Inherit: Same as input
      settings: AttributesFormatString=RT/Vm
  Prod1 : Product  OutDataTypeStr=single  RndMeth=Simplest
  Prod2 : Product  Inputs=3  OutDataTypeStr=single
  Prod3 : Product  Inputs=4  OutDataTypeStr=single
  Prod4 : Product  Inputs=4  OutDataTypeStr=single
  Prod5 : Product  OutDataTypeStr=Inherit: Inherit via back propagation  RndMeth=Simplest
  Sum1 : Sum  Inputs=|+-  OutDataTypeStr=single  RndMeth=Simplest  InputSameDT=on
  Sum2 : Sum  OutDataTypeStr=Inherit: Inherit via back propagation  InputSameDT=on
  Sum3 : Sum  Inputs=++++  OutDataTypeStr=single  InputSameDT=on
  UnitDelay1 : UnitDelay  InitialCondition=98200  SampleTime=-1  StateName=air_estimate
      settings: AttributesFormatString=p0 = %<InitialCondition> (bar)
  down_scale : Subsystem
      settings: AttributesFormatString=%<MemberBlocks>
  down_scale1 : Subsystem
      settings: AttributesFormatString=%<MemberBlocks>
  down_scale10 : Subsystem
      settings: AttributesFormatString=%<MemberBlocks>
  down_scale11 : Subsystem
      settings: AttributesFormatString=%<MemberBlocks>
  down_scale12 : Subsystem
      settings: AttributesFormatString=%<MemberBlocks>
  down_scale13 : Subsystem
      settings: AttributesFormatString=%<MemberBlocks>
  down_scale14 : Subsystem
      settings: AttributesFormatString=%<MemberBlocks>
  down_scale2 : Subsystem
      settings: AttributesFormatString=%<MemberBlocks>
  down_scale3 : Subsystem
      settings: AttributesFormatString=%<MemberBlocks>
  down_scale4 : Subsystem
      settings: AttributesFormatString=%<MemberBlocks>
  down_scale5 : Subsystem
      settings: AttributesFormatString=%<MemberBlocks>
  down_scale7 : Subsystem
      settings: AttributesFormatString=%<MemberBlocks>
  down_scale9 : Subsystem
      settings: AttributesFormatString=%<MemberBlocks>
  fb_sat : Scope
      settings: TimeRange=50  YMin=52.5  YMax=97.5  SaveName=ScopeData19
  fb_sat1 : Scope
      settings: TimeRange=50  YMin=810  YMax=895  SaveName=ScopeData20
  estimated_cyl_air_flow_gps : Outport
  wires:
  Constant5/1 -> Prod4/4
  Constant4/1 -> Prod3/4
  Constant3/1 -> Prod2/3
  Prod2/1 -> down_scale/1(In1)
  Constant2/1 -> down_scale1/1(In1)
  Sum1/1 -> Gain/1
  Gain/1 -> Prod1/1
  Sum2/1 -> UnitDelay1/1
  Constant1/1 -> Prod1/2
  down_scale5/1(Out1) -> Sum2/1
  down_scale/1(Out1) -> down_scale10/1(In1)
  Prod1/1 -> fb_sat1/1, down_scale5/1(In1)
  down_scale9/1(Out1) -> down_scale12/1(In1)
  Sum3/1 -> Sum1/2, estimated_cyl_air_flow_gps/1, fb_sat/1
  UnitDelay1/1 -> down_scale7/1(In1), Sum2/2
  engine_speed_radps/1 -> Prod5/2, Prod5/1, down_scale14/1(In1), Prod2/2
  down_scale7/1(Out1) -> down_scale2/1(In1), down_scale4/1(In1), Prod4/3, Prod2/1
  down_scale1/1(Out1) -> Sum3/1
  down_scale10/1(Out1) -> Sum3/2
  down_scale11/1(Out1) -> Sum3/3
  down_scale12/1(Out1) -> Sum3/4
  Prod3/1 -> down_scale3/1(In1)
  Constant6/1 -> Prod4/2
  Prod5/1 -> down_scale13/1(In1)
  down_scale13/1(Out1) -> Prod4/1
  Prod4/1 -> down_scale9/1(In1)
  down_scale4/1(Out1) -> Prod3/2
  down_scale2/1(Out1) -> Prod3/1
  down_scale14/1(Out1) -> Prod3/3
  down_scale3/1(Out1) -> down_scale11/1(In1)
  throttle_flow_gps/1 -> Sum1/1

== system AbstractFuelControl_M1_FP/Model 1/AF_Controller/fuel_controller/fuel_controller_10ms/down_scale1 ==
  In1 : Inport
  Constant8 : Constant  Value=100  OutDataTypeStr=Inherit: Inherit via back propagation  SampleTime=-1
      settings: AttributesFormatString=Value = %<Value>
  Divide2 : Product  Inputs=*/  OutDataTypeStr=single
  Out1 : Outport
  wires:
  Constant8/1 -> Divide2/2
  Divide2/1 -> Out1/1
  In1/1 -> Divide2/1

== system AbstractFuelControl_M1_FP/Model 1/AF_Controller/fuel_controller/fuel_controller_10ms/down_scale2 ==
  In1 : Inport
  Constant8 : Constant  OutDataTypeStr=single  SampleTime=-1
      settings: AttributesFormatString=Value = %<Value>
  Divide2 : Product  Inputs=*/  OutDataTypeStr=Inherit: Inherit via back propagation
  Out1 : Outport
  wires:
  Constant8/1 -> Divide2/2
  Divide2/1 -> Out1/1
  In1/1 -> Divide2/1

== system AbstractFuelControl_M1_FP/Model 1/AF_Controller/fuel_controller/fuel_controller_10ms/down_scale4 ==
  In1 : Inport
  Constant8 : Constant  Value=100  OutDataTypeStr=single  SampleTime=-1
      settings: AttributesFormatString=Value = %<Value>
  Divide2 : Product  Inputs=*/  OutDataTypeStr=Inherit: Inherit via back propagation
  Out1 : Outport
  wires:
  Constant8/1 -> Divide2/2
  Divide2/1 -> Out1/1
  In1/1 -> Divide2/1

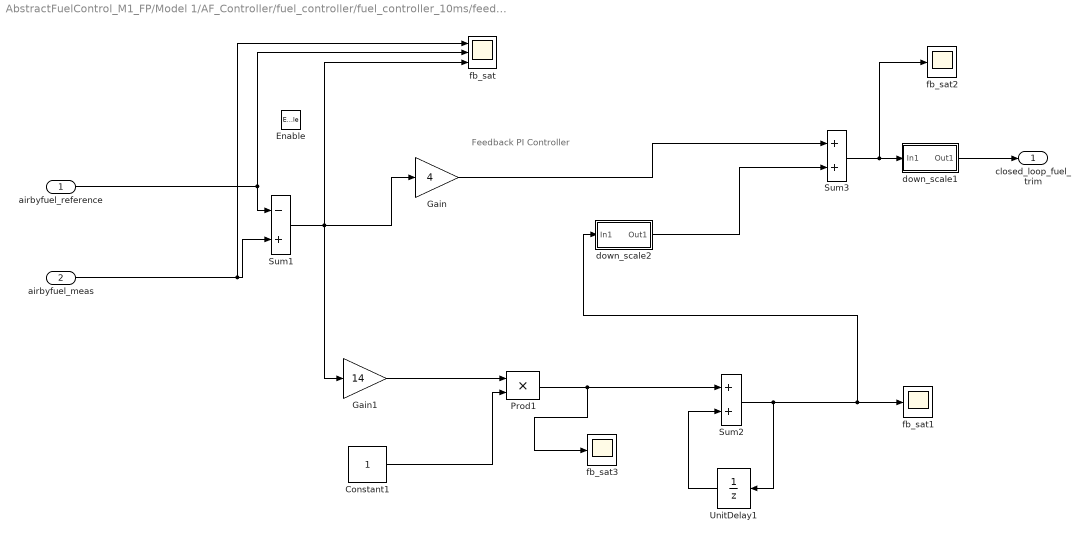
== system AbstractFuelControl_M1_FP/Model 1/AF_Controller/fuel_controller/fuel_controller_10ms/feedback_PI_controller ==
  note: Feedback PI Controller
  airbyfuel_reference : Inport
  airbyfuel_meas : Inport  Port=2
  Enable : EnablePort
  Constant1 : Constant  OutDataTypeStr=Inherit: Inherit via back propagation  SampleTime=-1
      settings: AttributesFormatString=Sample Time [s]
  Gain : Gain  Gain=4  OutDataTypeStr=single  RndMeth=Simplest  SaturateOnIntegerOverflow=on  ParamDataTypeStr=Inherit: Same as input
      settings: AttributesFormatString=Proportional Gain
  Gain1 : Gain  Gain=14  OutDataTypeStr=single  RndMeth=Simplest  ParamDataTypeStr=Inherit: Same as input
      settings: AttributesFormatString=Integral Gain
  Prod1 : Product  OutDataTypeStr=single
  Sum1 : Sum  Inputs=-+  OutDataTypeStr=Inherit: Inherit via back propagation  InputSameDT=on
  Sum2 : Sum  OutDataTypeStr=Inherit: Inherit via back propagation  InputSameDT=on
  Sum3 : Sum  AccumDataTypeStr=fixdt(1,32,0)  OutDataTypeStr=Inherit: Inherit via back propagation  InputSameDT=on
  UnitDelay1 : UnitDelay  SampleTime=-1  StateName=pi
      settings: AttributesFormatString=Initial Value = 0
  down_scale1 : Subsystem
      settings: AttributesFormatString=%<MemberBlocks>
  down_scale2 : Subsystem
      settings: AttributesFormatString=%<MemberBlocks>
  fb_sat : Scope  NumInputPorts=3
      settings: TimeRange=50  YMin=147700~139650~700  YMax=148300~154350~1300  SaveName=ScopeData13
  fb_sat1 : Scope
      settings: TimeRange=50  YMin=-500  YMax=350  SaveName=ScopeData14
  fb_sat2 : Scope
      settings: TimeRange=50  YMin=-100  YMax=1700  SaveName=ScopeData15
  fb_sat3 : Scope
      settings: TimeRange=45  YMin=-15  YMax=30  SaveName=ScopeData16
  closed_loop_fuel_trim : Outport
  wires:
  Gain/1 -> Sum3/1
  Constant1/1 -> Prod1/2
  UnitDelay1/1 -> Sum2/2
  Sum3/1 -> fb_sat2/1, down_scale1/1(In1)
  down_scale1/1(Out1) -> closed_loop_fuel_trim/1
  airbyfuel_reference/1 -> fb_sat/2, Sum1/1
  airbyfuel_meas/1 -> fb_sat/1, Sum1/2
  Sum1/1 -> fb_sat/3, Gain1/1, Gain/1
  Gain1/1 -> Prod1/1
  Sum2/1 -> down_scale2/1(In1), fb_sat1/1, UnitDelay1/1
  Prod1/1 -> Sum2/1, fb_sat3/1
  down_scale2/1(Out1) -> Sum3/2

== system AbstractFuelControl_M1_FP/Model 1/AF_Controller/fuel_controller/fuel_controller_10ms/feedforward_controller ==
  note: Feedforward Controller
  estimated_cyl_air_flow_gps : Inport
  airbyfuel_reference : Inport  Port=2
  Gain1 : Gain  Gain=100  OutDataTypeStr=Inherit: Inherit via back propagation  ParamDataTypeStr=Inherit: Same as input
      settings: AttributesFormatString=up_scale
  Product : Product  Inputs=*/  OutDataTypeStr=single
  fb_sat1 : Scope  NumInputPorts=3
      settings: TimeRange=30.1  YMin=38~555000~139.65  YMax=45~655000~154.35  SaveName=ScopeData18
  desired_fuel_mass_gps : Outport
  wires:
  airbyfuel_reference/1 -> fb_sat1/3, Product/2
  estimated_cyl_air_flow_gps/1 -> Gain1/1
  Gain1/1 -> fb_sat1/2, Product/1
  Product/1 -> fb_sat1/1, desired_fuel_mass_gps/1

== system AbstractFuelControl_M1_FP/Model 1/AF_Controller/fuel_controller/fuel_controller_mode_10ms/normal_mode_detection ==
  note: Normal Mode Detection (Cold Start to Normal)
  note: NOTE: For first 10 seconds, controller uses only feedforward control to ignore the initialization issue.
  Logical Operator : Logic  Operator=OR  OutDataTypeStr=boolean
  Relational Operator : RelationalOperator  OutDataTypeStr=boolean
  Scope : Scope
      settings: TimeRange=0.06737519927813551  YMin=1  YMax=1  SaveName=ScopeData2
  Sum : Sum
  Unit Delay1 : UnitDelay  SampleTime=-1  StateName=normal_mode_detect_1
      settings: AttributesFormatString=Initial Value = 0
  Unit Delay2 : UnitDelay  SampleTime=-1  StateName=normal_mode_detect_1
      settings: AttributesFormatString=Initial Value = 0
  normal_mode_start_sec : Constant  Value=1000  OutDataTypeStr=Inherit: Inherit via back propagation  SampleTime=-1
      settings: AttributesFormatString=Normal Mode Start Time (s)
  sampling_sec : Constant  OutDataTypeStr=Inherit: Inherit via back propagation  SampleTime=-1
      settings: AttributesFormatString=Sample Time (s)
  ud2 : ToWorkspace  VariableName=ud2  SampleTime=-1  SaveFormat=Timeseries
      settings: MaxDataPoints=1
  normal_on : Outport
  wires:
  Relational Operator/1 -> Logical Operator/1
  normal_mode_start_sec/1 -> Relational Operator/2
  Unit Delay1/1 -> Logical Operator/2
  Logical Operator/1 -> Unit Delay1/1, Scope/1, ud2/1, normal_on/1
  sampling_sec/1 -> Sum/2
  Unit Delay2/1 -> Sum/1
  Sum/1 -> Relational Operator/1, Unit Delay2/1

== system AbstractFuelControl_M1_FP/Model 1/AF_Controller/fuel_controller/fuel_controller_mode_10ms/power_mode_detection ==
  note: Power Mode Detection
  throttle_angle : Inport
  Constant : Constant  Value=500  OutDataTypeStr=Inherit: Inherit via back propagation
      settings: AttributesFormatString=Base
  Constant1 : Constant  Value=200  OutDataTypeStr=Inherit: Inherit via back propagation
      settings: AttributesFormatString=Hysteresis
  Relational Operator1 : RelationalOperator  OutDataTypeStr=boolean
  Sum : Sum
  Switch : Switch  Criteria=u2 ~= 0
  Unit Delay1 : UnitDelay  SampleTime=-1  StateName=power_mode_detect
      settings: AttributesFormatString=Initial Value = 0
  power_on : Outport
  wires:
  Sum/1 -> Switch/3
  Constant1/1 -> Sum/2
  Constant/1 -> Switch/1, Sum/1
  throttle_angle/1 -> Relational Operator1/1
  Switch/1 -> Relational Operator1/2
  Unit Delay1/1 -> Switch/2
  Relational Operator1/1 -> power_on/1, Unit Delay1/1

== system AbstractFuelControl_M1_FP/Model 1/AF_Controller/fuel_controller/fuel_controller_mode_10ms/sensor_failure_detection ==
  note: A/F Sensor Failuer Detection
  airbyfuel_meas : Inport
  Logical Operator : Logic  Operator=OR  OutDataTypeStr=boolean
  Relational Operator : RelationalOperator  Operator=<=  OutDataTypeStr=boolean
  Unit Delay : UnitDelay  SampleTime=-1  StateName=sensor_fail_detect
      settings: AttributesFormatString=Initial Value = 0
  threshold : Constant  Value=-10  OutDataTypeStr=Inherit: Inherit via back propagation
  fail_on : Outport
  wires:
  Relational Operator/1 -> Logical Operator/1
  threshold/1 -> Relational Operator/2
  Unit Delay/1 -> Logical Operator/2
  Logical Operator/1 -> Unit Delay/1, fail_on/1
  airbyfuel_meas/1 -> Relational Operator/1

== system AbstractFuelControl_M1_FP/Model 1/AF_Controller/fuel_controller/fuel_controller_10ms/air_estimation/down_scale ==
  In1 : Inport
  Constant8 : Constant  Value=10  OutDataTypeStr=Inherit: Inherit via back propagation  SampleTime=-1
      settings: AttributesFormatString=Value = %<Value>
  Divide2 : Product  Inputs=*/  OutDataTypeStr=Inherit: Inherit via back propagation
  Out1 : Outport
  wires:
  Constant8/1 -> Divide2/2
  Divide2/1 -> Out1/1
  In1/1 -> Divide2/1

== system AbstractFuelControl_M1_FP/Model 1/AF_Controller/fuel_controller/fuel_controller_10ms/air_estimation/down_scale1 ==
  In1 : Inport
  Constant8 : Constant  Value=100000  OutDataTypeStr=Inherit: Inherit via back propagation  SampleTime=-1
      settings: AttributesFormatString=Value = %<Value>
  Divide2 : Product  Inputs=*/  OutDataTypeStr=Inherit: Inherit via back propagation
  Out1 : Outport
  wires:
  Constant8/1 -> Divide2/2
  Divide2/1 -> Out1/1
  In1/1 -> Divide2/1

== system AbstractFuelControl_M1_FP/Model 1/AF_Controller/fuel_controller/fuel_controller_10ms/air_estimation/down_scale10 ==
  In1 : Inport
  Constant8 : Constant  Value=100000  OutDataTypeStr=Inherit: Inherit via back propagation  SampleTime=-1
      settings: AttributesFormatString=Value = %<Value>
  Divide2 : Product  Inputs=*/  OutDataTypeStr=Inherit: Inherit via back propagation
  Out1 : Outport
  wires:
  Constant8/1 -> Divide2/2
  Divide2/1 -> Out1/1
  In1/1 -> Divide2/1

== system AbstractFuelControl_M1_FP/Model 1/AF_Controller/fuel_controller/fuel_controller_10ms/air_estimation/down_scale11 ==
  In1 : Inport
  Constant8 : Constant  Value=100  OutDataTypeStr=Inherit: Inherit via back propagation  SampleTime=-1
      settings: AttributesFormatString=Value = %<Value>
  Divide2 : Product  Inputs=*/  OutDataTypeStr=Inherit: Inherit via back propagation
  Out1 : Outport
  wires:
  Constant8/1 -> Divide2/2
  Divide2/1 -> Out1/1
  In1/1 -> Divide2/1
